simulink model "LQR2020a"  (R2020a)
settings: Solver=FixedStepAuto  StartTime=0.0  StopTime=300  FixedStep=0.05  RelTol=1e-3
InitFcn:
  | startPose=[0,0,48]
StopFcn:
  | load('NewBaiYunPathDown6_13.mat')
  | n=1;
  | x0=0;
  | y0=0;
  | lng0 = BaiYunEmpty(2,1);
  | lat0 = BaiYunEmpty(1,1);
  | x1=[];
  | y1=[];
  | head=[];
  | nn = length(BaiYunEmpty(1,:));
  | while (n<nn)
  | lng2 = BaiYunEmpty(2,n);
  | lat2 = BaiYunEmpty(1,n);
  | head2 = BaiYunEmpty(3,n);
  | temp_x=(lng2-lng0)*111700*cos(lat2/180*pi);
  | temp_y=(lat2-lat0)*111700;
  | x1(n) = x0 + temp_x;
  | y1(n) = y0 + temp_y;
  | head(n)=head2;
  | n = n+1;
  | end
  | figure(1);
  | plot(x1,y1,'+r',out.v2(:,1),out.v2(:,2),'+k',out.v3(:,1),out.v3(:,2),'+b');
libraries: simulink x21, simulink_extras x4, drivingvehiclecontroller x2, vehdynlibsteering x2, autolibshared x2
(part 2 of 2)

== matlab function LQR2020a/Lateral_Control_Simulation-2/path_process1 ==
  data: curpoint input; speed_actual input; d output; v_tra output; steer_angle_feedback output; steer_angle output; steer_angle_feedforwardterm output; curvehhead input; curwheelangle input; curryawrate input; matrix_k_ output; matrix_temp1 output; lateral_error output; heading_error output
function [d,v_tra,steer_angle_feedback,steer_angle,steer_angle_feedforwardterm,matrix_k_,matrix_temp1,lateral_error,heading_error]  = fcn(curpoint,speed_actual,curvehhead,curwheelangle,curryawrate)
PREDICT_TIME_CTL=1.2;        %%s
WHEEL_BASE=5.635;            %%m
R2D=57.2957805;
D2R=0.0174533;
STEER_DELAY_TIME=0.0;        %%s
ANGLE_CORRECT_PARAM=1.5;

cf_ = 4e4;
cr_ = 6e4;
mass_=25000;
iz_=60000;
lf_ = 2.55;
lr_ = 2.675;
ts_ = 0.05;
lqr_eps_ = 0.01;
lqr_max_iteration_ = 150;
wheelbase_=5.225;

speed_actual=max(1,speed_actual);

matrix_a_ = [0,1,0,0;
             0,0,(cf_ + cr_) / mass_,0;
             0,0,0,1;
             (lf_ * cf_ - lr_ * cr_) / iz_,0,0,0;];
matrix_a_coeff_ = [0,0,0,0;
                   0,-(cf_ + cr_)/mass_,0,(lr_ * cr_ - lf_ * cf_) / mass_;
                   0,0,0,1;
                   0,(lr_ * cr_ - lf_ * cf_) / iz_,0,-1.0 * (lf_ * lf_ * cf_ + lr_ * lr_ * cr_) / iz_;];
matrix_b_ = [0;
             cf_ / mass_;
             0;
             lf_ * cf_ / iz_;];
matrix_bd_ = matrix_b_ * ts_;

matrix_state_ = zeros(4, 1);
matrix_k_ = zeros(1,4);
matrix_r_ = eye(1,1);
matrix_q_ = zeros(4,4);
matrix_q_(1, 1)=20;
matrix_q_(3, 3)=2; 
matrix_q_updated_ = matrix_q_;

%载入路径文件
Q = load('NewBaiYunPathDown6_13.mat');
dis_last = 100000;
abc=1;
abc_last = 1;
n=1;
x0=0;
y0=0;
lng0 = Q.BaiYunEmpty(2,1);
lat0 = Q.BaiYunEmpty(1,1);
temp_n = length(Q.BaiYunEmpty(1,:));

%%计算关键点
while (n<temp_n)    
lng2 = Q.BaiYunEmpty(2,n);
lat2 = Q.BaiYunEmpty(1,n);
temp_x=(lng2-lng0)*111700*cos(lat2/180*pi);
temp_y=(lat2-lat0)*111700;    
x1 = x0 + temp_x;
y1 = y0 + temp_y;
x2=curpoint(1);
y2=curpoint(2);
    dis=sqrt((x1-x2)^2+(y1-y2)^2);
    if(dis<dis_last)
        abc=n;
        dis_last = dis;
    else
        abc=abc_last;
    end
abc_last = abc;
n = n+1;
end
keypointlist = abc;%得到关键点id
%%计算关键点和关键点前一点的xy
key_x=(Q.BaiYunEmpty(2,keypointlist)-lng0)*111700*cos(Q.BaiYunEmpty(1,keypointlist)/180*pi);
key_y=(Q.BaiYunEmpty(1,keypointlist)-lat0)*111700; 
key_theta=Q.BaiYunEmpty(3,keypointlist);
key_x1=(Q.BaiYunEmpty(2,keypointlist+1)-lng0)*111700*cos(Q.BaiYunEmpty(1,keypointlist+1)/180*pi);
key_y1=(Q.BaiYunEmpty(1,keypointlist+1)-lat0)*111700; 
key_delta_x = key_x - curpoint(1);
key_delta_y = key_y - curpoint(2);
key_delta_x1 = key_x1 - curpoint(1);
key_delta_y1 = key_y1 - curpoint(2);
%%计算横向偏差
dis1 = sqrt((key_delta_x1)^2+(key_delta_y1)^2);
dis2 = sqrt((key_x1-key_x)^2+(key_y1-key_y)^2);
area = 1/4*sqrt((dis_last+dis1+dis2)*(dis_last+dis1-dis2)*(dis_last+dis2-dis1)*(dis1+dis2-dis_last));
if(dis2>=0.01)
    d=2.0*area/dis2;
else
    d=dis_last;
end      

if(key_delta_x>-0.0001&&key_delta_x<0.0001)
    if(key_delta_y>0)
        key_point_direction=0;
    else
        key_point_direction=180;
    end    
else    
   key_point_direction = atan(key_delta_y / key_delta_x) / pi*180;
    if (key_delta_x > 0) 
        key_point_direction = 90 - key_point_direction;
    else
        key_point_direction = 270 - key_point_direction;
    end
end

%%计算关键点附近曲率
n=1;
Larc=0;
while(n<=5)
Larc_add = getDistance(Q.BaiYunEmpty(1,keypointlist),Q.BaiYunEmpty(2,keypointlist),Q.BaiYunEmpty(1,keypointlist+n),Q.BaiYunEmpty(2,keypointlist+n));    
Larc = Larc+Larc_add;
n=n+1;
end
delta_head = Q.BaiYunEmpty(3,keypointlist+5)-Q.BaiYunEmpty(3,keypointlist);
kappa = delta_head*D2R/Larc;
%%%%%%%%%%%%%%%%%%%

%%apollo横向偏差计算
dx_apo = curpoint(1) - key_x;
dy_apo = curpoint(2) - key_y;
cos_target_heading = cos(key_theta*D2R);
sin_target_heading = sin(key_theta*D2R);
lateral_error = cos_target_heading * dy_apo - sin_target_heading * dx_apo;
heading_error = key_theta - curvehhead;
lateral_error_dot = speed_actual*sin(heading_error);
heading_error_rate = kappa*speed_actual - curryawrate;

matrix_state_(1, 1) = lateral_error;
matrix_state_(2, 1) = lateral_error_dot;
matrix_state_(3, 1) = heading_error;
matrix_state_(4, 1) = heading_error_rate;

matrix_a_(2, 2) = matrix_a_coeff_(2, 2) / speed_actual;
matrix_a_(2, 4) = matrix_a_coeff_(2, 4) / speed_actual;
matrix_a_(4, 2) = matrix_a_coeff_(4, 2) / speed_actual;
matrix_a_(4, 4) = matrix_a_coeff_(4, 4) / speed_actual;
matrix_i = eye(4,4);
matrix_ad_ = inv(matrix_i - ts_ * 0.5 * matrix_a_)*(matrix_i + ts_ * 0.5 * matrix_a_);

matrix_k_ = SolveLQRProblem(matrix_ad_, matrix_bd_, matrix_q_updated_,matrix_r_, lqr_eps_, lqr_max_iteration_);
matrix_k_(1,2)=0;

matrix_k_(1,4)=0;
matrix_temp1 = matrix_k_ * matrix_state_;
steer_angle_feedback = matrix_temp1;

kv = lr_ * mass_ / 2 / cf_ / wheelbase_ - lf_ * mass_ / 2 / cr_ / wheelbase_;

steer_angle_feedforwardterm =R2D*(wheelbase_ * kappa + kv * speed_actual * speed_actual * kappa - matrix_k_(1, 3) *(lr_ * kappa -lf_ * mass_ * speed_actual * speed_actual * kappa / 2 / cr_ / wheelbase_));
steer_angle = steer_angle_feedback+steer_angle_feedforwardterm;
v_tra = Q.BaiYunEmpty(4,keypointlist);

end

function result_angle = getAngleByTwoGps(lat1, lng1, lat2, lng2)
R2D=57.2957805;
D2R=0.0174533;
dx = (lng2 - lng1) * 111700 *cos(lat1*D2R);
dy = (lat2 - lat1) * 111700;

result_angle = atan2(dx,dy)*R2D;%%计算与y轴正方向的夹角(-180~180)
if(result_angle <0)
    result_angle = 360+result_angle;
end
end

function K = SolveLQRProblem(A,B,Q,R,tolerance,max_num_iteration)
AT = A';
BT = B';
P = Q;
num_iteration = 0;
diff = 10000;
while(num_iteration < max_num_iteration && diff > tolerance)
    P_next =AT * P * A - AT * P * B * inv(R + BT * P * B) * BT * P * A + Q;
    diff = max(max(abs(P_next - P)));
    P=P_next;
    num_iteration=num_iteration+1;
end
K = inv(R + BT * P * B) * BT * P * A;
end

function Dis = getDistance(lat1,lng1,lat2,lng2)

    x=abs(lng1-lng2)*111700*cos(lat1/180*3.141592653589793);
    y=abs(lat1-lat2)*111700;

    Dis=sqrt(x*x+y*y);
end
